simulink model "APR_AWGN_histogram_stats_2020b"  (R2020b)
settings: Solver=VariableStepAuto  StartTime=0.0  StopTime=15.0  RelTol=1e-3
undefined symbols (not defined in the file): Fs, ip, usb
libraries: visionstatistics x3, plutoradiolib x1, dspsigops x1, dspstat3 x1
settings Model: Creator=14083  LastModifiedBy=14083

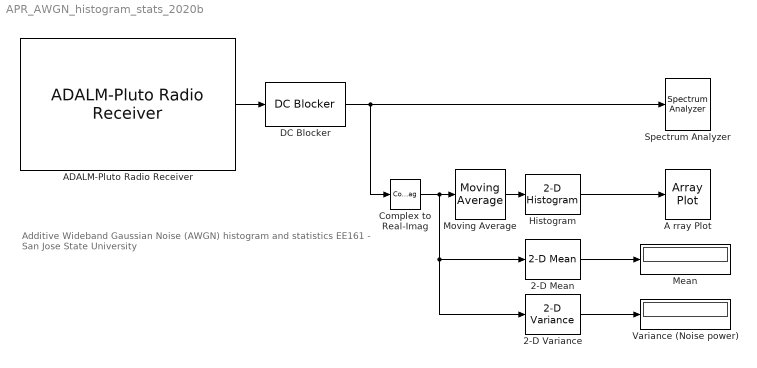
== system APR_AWGN_histogram_stats_2020b ==
  note: Additive Wideband Gaussian Noise (AWGN) histogram
      | and statistics
      | EE161 - San Jose State University
  2-D Mean : visionstatistics/2-D Mean  run=off  reset_popup=None  directionMode=Entire input  dimension=1  treatSBRowAsCol=on  outputLastDataTypeStr=Inherit: Same as accumulator  accumMode=Binary point scaling  accumWordLength=32  accumFracLength=0  accumLastDataTypeStr=fixdt([],32,0)  roiEnable=off  roiType=Rectangles  roiPortion=Entire ROI  roiOutput=Individual statistics for each ROI  roiFlag=off  roundingMode=Floor  overflowMode=off  accumDataTypeStr=fixdt([],32,0)  outputDataTypeStr=Inherit: Same as accumulator  outputMin=[]  outputMax=[]
      settings: SourceProductBaseCode=VP
  2-D Variance : visionstatistics/2-D Variance  run=off  reset_popup=None  directionMode=Entire input  dimension=1  treatSBRowAsCol=on  roiEnable=off  roiType=Rectangles  roiPortion=Entire ROI  roiOutput=Individual statistics for each ROI  roiFlag=off  roundingMode=Floor  overflowMode=off  prodOutputMode=Binary point scaling  prodOutputWordLength=32  prodOutputFracLength=0  prodOutputSlope=2^0  memorySlope=2^-30  accumSlope=2^-32  outputSlope=2^-32
      settings: SourceProductBaseCode=VP
  "A rray Plot " : ArrayPlot
  ADALM-Pluto Radio Receiver : plutoradiolib/ADALM-Pluto Radio Receiver  RadioID=usb:0  uri=ip:10.0.0.200  CenterFrequencySource=Dialog  CenterFrequency=900e6  GainSource=AGC Slow Attack  GainSourceBlock=Dialog  Gain=0  ChannelMapping=1  BasebandSampleRate=1e6  OutputDataType=single  SamplesPerFrame=10000  OverflowOutputPort=off  EnableBurstMode=off  NumFramesInBurst=1  ShowAdvancedProperties=off  UseCustomFilter=off  filtPathRates=[737280000 11520000 3840000 1920000 960000 240000]  filtCoefficients=[-192 82 85 -215 228 -102 -110 290 -318 145 160 -426 471 -215 -238 633 -697 318 349 -923 1009 -457 -498 1309 -1423 640 693 -1812 1959 -876 -945 2458 -2647 1180 1268 -3290 3534 -1572 -1688 4375 -4698 2091 2247 -5836 6284 -2807 -3031 7918 -8588 3870 4225 -11182 12324 -5662 -6330 17255 -19735 9507 11312 -33568 43355 -25227 -42139 305542 305542 -42139 -25227 43355 -33568 11312 9507 -19735 17255 -6330 -5662 12324 -11182 4225 3870 -8588 7918 -3031 -2807 6284 -5836 2247 2091 -4698 4375 -1688 -1572 3534 -3290 1268 1180 -2647 2458 -945 -876 1959 -1812 693 640 -1423 1309 -498 -457 1009 -923 349 318 -697 633 -238 -215 471 -426 160 145 -318 290 -110 -102 228 -215 85 82 -192]  filtCoefficientSize=128  filtDecimInterpFactor=4  filtGain=-12  filtRFBandwidth=18000000  filterConfigStruct=struct()  EnableQuadratureCorrection=on  EnableRFDCCorrection=on  EnableBasebandDCCorrection=on  FrequencyCorrection=0  OverrideSampleTime=off  SampleTime=0.02  DataTimeout=Inf  ENSMPinControlMode=None  BISTLoopbackMode=Disabled  BISTToneInject=Disabled  BISTSignalGen=PRBS  BISTToneFreq=Fs/32  BISTToneLevel=0
      settings: SourceProductBaseCode=PLUTO
  Complex to Real-Imag : ComplexToRealImag  Output=Real
  DC Blocker : dspsigops/DC Blocker  Algorithm=FIR  NormalizedBandwidth=0.001  Length=128  Order=6  SimulateUsing=Code generation
      settings: SourceProductName=DSP System Toolbox
  Histogram : visionstatistics/2-D Histogram  umin=-0.0003  umax=0.0003  nbins=50  operateOver=Each column  normalized=on  run=off  reset=on  trigtype=None  Dimension=1  colComp=on  roundingMode=Floor  overflowMode=off
      settings: SourceProductBaseCode=VP
  Mean : Display
  Moving Average : dspstat3/Moving Average  Method=Sliding window  ForgettingFactorPort=off  SpecifyWindowLength=on  WindowLength=22  ForgettingFactor=0.9  SimulateUsing=Code generation
  "Spectrum Analyzer " : SpectrumAnalyzer
  Variance (Noise power) : Display
  wires:
  ADALM-Pluto Radio Receiver/1 -> DC Blocker/1
  DC Blocker/1 -> Complex to Real-Imag/1, "Spectrum Analyzer "/1
  Moving Average/1 -> Histogram/1
  Histogram/1 -> "A rray Plot "/1
  2-D Mean/1 -> Mean/1
  Complex to Real-Imag/1 -> 2-D Variance/1, 2-D Mean/1, Moving Average/1
  2-D Variance/1 -> Variance (Noise power)/1
